simulink model "chap04_CA1"  (R2021a)
settings: Solver=FixedStepDiscrete  StartTime=0.0  StopTime=30  FixedStep=0.001  RelTol=1e-3
undefined symbols (not defined in the file): DiscIntNeverNeededParam
libraries: simulink x4
(part 4 of 4)

== system chap04_CA1/Subsystem/Subsystem13/Subsystem7/Subsystem12 ==
  xx2 : Inport
  xx1 : Inport  Port=2
  xx4 : Inport  Port=3
  xx6 : Inport  Port=4
  Add1 : Sum  Inputs=-+
  Add2 : Sum  Inputs=+-
  Add4 : Sum  Inputs=-+
  Add5 : Sum  Inputs=+++
  Constant3 : Constant  Value=0.5
  Constant4 : Constant  Value=1.0
  Constant5 : Constant  Value=1.5
  Product3 : Product
  Product4 : Product
  Product5 : Product
  p2x : Outport
  wires:
  Product4/1 -> Add5/2
  Product5/1 -> Add5/3
  Constant3/1 -> Product4/1
  Add4/1 -> Product4/2
  xx2/1 -> Add1/2, Add4/2, Add2/1
  Constant4/1 -> Product5/2
  Add2/1 -> Product5/1
  xx4/1 -> Add4/1
  xx1/1 -> Add2/2
  xx6/1 -> Add1/1
  Constant5/1 -> Product3/1
  Add1/1 -> Product3/2
  Product3/1 -> Add5/1
  Add5/1 -> p2x/1

== system chap04_CA1/Subsystem/Subsystem13/Subsystem7/Subsystem7 ==
  vy2 : Inport
  vy1 : Inport  Port=2
  vy4 : Inport  Port=3
  vy6 : Inport  Port=4
  Add6 : Sum  Inputs=-+
  Add7 : Sum  Inputs=+-
  Add8 : Sum  Inputs=-+
  Add9 : Sum  Inputs=+++
  Constant3 : Constant  Value=0.5
  Constant4 : Constant  Value=1.0
  Constant5 : Constant  Value=1.5
  Product7 : Product
  Product8 : Product
  Product9 : Product
  p2y : Outport
  wires:
  Product8/1 -> Add9/2
  Product9/1 -> Add9/3
  Constant3/1 -> Product8/1
  Add8/1 -> Product8/2
  vy2/1 -> Add6/2, Add8/2, Add7/1
  Constant4/1 -> Product9/2
  Add7/1 -> Product9/1
  vy4/1 -> Add8/1
  vy1/1 -> Add7/2
  vy6/1 -> Add6/1
  Constant5/1 -> Product7/1
  Add6/1 -> Product7/2
  Product7/1 -> Add9/1
  Add9/1 -> p2y/1

== system chap04_CA1/Subsystem/Subsystem13/Subsystem7/Subsystem8 ==
  vz2 : Inport
  vz1 : Inport  Port=2
  vz4 : Inport  Port=3
  vz6 : Inport  Port=4
  Add6 : Sum  Inputs=-+
  Add7 : Sum  Inputs=+-
  Add8 : Sum  Inputs=-+
  Add9 : Sum  Inputs=+++
  Constant3 : Constant  Value=0.5
  Constant4 : Constant  Value=1.0
  Constant5 : Constant  Value=1.5
  Product7 : Product
  Product8 : Product
  Product9 : Product
  p2z : Outport
  wires:
  Product7/1 -> Add9/1
  Add6/1 -> Product7/2
  Constant5/1 -> Product7/1
  vz6/1 -> Add6/1
  vz1/1 -> Add7/2
  vz4/1 -> Add8/1
  Add7/1 -> Product9/1
  Constant4/1 -> Product9/2
  vz2/1 -> Add7/1, Add8/2, Add6/2
  Add8/1 -> Product8/2
  Constant3/1 -> Product8/1
  Product9/1 -> Add9/3
  Product8/1 -> Add9/2
  Add9/1 -> p2z/1

== system chap04_CA1/Subsystem/Subsystem13/Subsystem7/Subsystem9 ==
  vx2 : Inport
  vx1 : Inport  Port=2
  vx4 : Inport  Port=3
  vx6 : Inport  Port=4
  Add6 : Sum  Inputs=-+
  Add7 : Sum  Inputs=+-
  Add8 : Sum  Inputs=-+
  Add9 : Sum  Inputs=+++
  Constant3 : Constant  Value=0.5
  Constant4 : Constant  Value=1.0
  Constant5 : Constant  Value=1.5
  Product7 : Product
  Product8 : Product
  Product9 : Product
  p2x : Outport
  wires:
  Add9/1 -> p2x/1
  Product7/1 -> Add9/1
  Add6/1 -> Product7/2
  Constant5/1 -> Product7/1
  vx6/1 -> Add6/1
  vx1/1 -> Add7/2
  vx4/1 -> Add8/1
  Add7/1 -> Product9/1
  Constant4/1 -> Product9/2
  vx2/1 -> Add7/1, Add8/2, Add6/2
  Add8/1 -> Product8/2
  Constant3/1 -> Product8/1
  Product9/1 -> Add9/3
  Product8/1 -> Add9/2

== system chap04_CA1/Subsystem/Subsystem6/Subsystem/Subsystem3 ==
  xyk : Inport
  xy : Inport  Port=2
  Add4 : Sum  Inputs=-+
  exy : Outport
  wires:
  xy/1 -> Add4/1
  Add4/1 -> exy/1
  xyk/1 -> Add4/2

== system chap04_CA1/Subsystem/Subsystem6/Subsystem/Subsystem4 ==
  xzk : Inport
  xz : Inport  Port=2
  Add4 : Sum  Inputs=-+
  exz : Outport
  wires:
  xzk/1 -> Add4/2
  Add4/1 -> exz/1
  xz/1 -> Add4/1

== system chap04_CA1/Subsystem/Subsystem6/Subsystem/Subsystem5 ==
  xxk : Inport
  xx : Inport  Port=2
  Add4 : Sum  Inputs=-+
  exx : Outport
  wires:
  xxk/1 -> Add4/2
  Add4/1 -> exx/1
  xx/1 -> Add4/1

== system chap04_CA1/Subsystem/Subsystem6/Subsystem/Subsystem7 ==
  vyk : Inport
  vy : Inport  Port=2
  Add8 : Sum  Inputs=-+
  ey : Outport
  wires:
  Add8/1 -> ey/1
  vy/1 -> Add8/1
  vyk/1 -> Add8/2

== system chap04_CA1/Subsystem/Subsystem6/Subsystem/Subsystem8 ==
  vzk : Inport
  vz : Inport  Port=2
  Add8 : Sum  Inputs=-+
  ez : Outport
  wires:
  vzk/1 -> Add8/2
  vz/1 -> Add8/1
  Add8/1 -> ez/1

== system chap04_CA1/Subsystem/Subsystem6/Subsystem/Subsystem9 ==
  vxk : Inport
  vx : Inport  Port=2
  Add8 : Sum  Inputs=-+
  evx : Outport
  wires:
  vxk/1 -> Add8/2
  vx/1 -> Add8/1
  Add8/1 -> evx/1

== system chap04_CA1/Subsystem/Subsystem6/Subsystem7/Subsystem1 ==
  xy1 : Inport
  xy2 : Inport  Port=2
  xy3 : Inport  Port=3
  xy6 : Inport  Port=4
  Add1 : Sum  Inputs=-+
  Add2 : Sum  Inputs=+-
  Add4 : Sum  Inputs=-+
  Add5 : Sum  Inputs=+++
  Constant1 : Constant  Value=0.5
  Constant2 : Constant  Value=1.0
  Constant6 : Constant  Value=1.2
  Product3 : Product
  Product4 : Product
  Product5 : Product
  pxy : Outport
  wires:
  Product4/1 -> Add5/2
  Product5/1 -> Add5/3
  Constant1/1 -> Product4/1
  Add4/1 -> Product4/2
  xy1/1 -> Add1/2, Add4/2, Add2/1
  Constant2/1 -> Product5/2
  Add2/1 -> Product5/1
  Add5/1 -> pxy/1
  xy3/1 -> Add4/1
  xy2/1 -> Add2/2
  xy6/1 -> Add1/1
  Constant6/1 -> Product3/1
  Add1/1 -> Product3/2
  Product3/1 -> Add5/1

== system chap04_CA1/Subsystem/Subsystem6/Subsystem7/Subsystem2 ==
  xz1 : Inport
  xx2 : Inport  Port=2
  xz3 : Inport  Port=3
  xz6 : Inport  Port=4
  Add1 : Sum  Inputs=-+
  Add2 : Sum  Inputs=+-
  Add4 : Sum  Inputs=-+
  Add5 : Sum  Inputs=+++
  Constant1 : Constant  Value=0.5
  Constant2 : Constant  Value=1.0
  Constant6 : Constant  Value=1.2
  Product3 : Product
  Product4 : Product
  Product5 : Product
  pxz : Outport
  wires:
  Product3/1 -> Add5/1
  Add1/1 -> Product3/2
  Constant6/1 -> Product3/1
  xz6/1 -> Add1/1
  xx2/1 -> Add2/2
  xz3/1 -> Add4/1
  Add5/1 -> pxz/1
  Add2/1 -> Product5/1
  Constant2/1 -> Product5/2
  xz1/1 -> Add2/1, Add4/2, Add1/2
  Add4/1 -> Product4/2
  Constant1/1 -> Product4/1
  Product5/1 -> Add5/3
  Product4/1 -> Add5/2

== system chap04_CA1/Subsystem/Subsystem6/Subsystem7/Subsystem3 ==
  vy1 : Inport
  vy2 : Inport  Port=2
  vy3 : Inport  Port=3
  vy6 : Inport  Port=4
  Add6 : Sum  Inputs=-+
  Add7 : Sum  Inputs=+-
  Add8 : Sum  Inputs=-+
  Add9 : Sum  Inputs=+++
  Constant1 : Constant  Value=0.5
  Constant2 : Constant  Value=1.0
  Constant6 : Constant  Value=1.2
  Product7 : Product
  Product8 : Product
  Product9 : Product
  pvy : Outport
  wires:
  Product8/1 -> Add9/2
  Product9/1 -> Add9/3
  Constant1/1 -> Product8/1
  Add8/1 -> Product8/2
  vy1/1 -> Add6/2, Add8/2, Add7/1
  Constant2/1 -> Product9/2
  Add7/1 -> Product9/1
  vy3/1 -> Add8/1
  vy2/1 -> Add7/2
  vy6/1 -> Add6/1
  Constant6/1 -> Product7/1
  Add6/1 -> Product7/2
  Product7/1 -> Add9/1
  Add9/1 -> pvy/1

== system chap04_CA1/Subsystem/Subsystem6/Subsystem7/Subsystem4 ==
  vz1 : Inport
  vz2 : Inport  Port=2
  vz3 : Inport  Port=3
  vz6 : Inport  Port=4
  Add6 : Sum  Inputs=-+
  Add7 : Sum  Inputs=+-
  Add8 : Sum  Inputs=-+
  Add9 : Sum  Inputs=+++
  Constant1 : Constant  Value=0.5
  Constant2 : Constant  Value=1.0
  Constant6 : Constant  Value=1.2
  Product7 : Product
  Product8 : Product
  Product9 : Product
  pvz : Outport
  wires:
  Add9/1 -> pvz/1
  Product7/1 -> Add9/1
  Add6/1 -> Product7/2
  Constant6/1 -> Product7/1
  vz6/1 -> Add6/1
  vz2/1 -> Add7/2
  vz3/1 -> Add8/1
  Add7/1 -> Product9/1
  Constant2/1 -> Product9/2
  vz1/1 -> Add7/1, Add8/2, Add6/2
  Add8/1 -> Product8/2
  Constant1/1 -> Product8/1
  Product9/1 -> Add9/3
  Product8/1 -> Add9/2

== system chap04_CA1/Subsystem/Subsystem6/Subsystem7/Subsystem5 ==
  vx1 : Inport
  vx2 : Inport  Port=2
  vx3 : Inport  Port=3
  vx6 : Inport  Port=4
  Add6 : Sum  Inputs=-+
  Add7 : Sum  Inputs=+-
  Add8 : Sum  Inputs=-+
  Add9 : Sum  Inputs=+++
  Constant1 : Constant  Value=0.5
  Constant2 : Constant  Value=1.0
  Constant6 : Constant  Value=1.2
  Product7 : Product
  Product8 : Product
  Product9 : Product
  pvx : Outport
  wires:
  Add9/1 -> pvx/1
  Product7/1 -> Add9/1
  Add6/1 -> Product7/2
  Constant6/1 -> Product7/1
  vx6/1 -> Add6/1
  vx2/1 -> Add7/2
  vx3/1 -> Add8/1
  Add7/1 -> Product9/1
  Constant2/1 -> Product9/2
  vx1/1 -> Add7/1, Add8/2, Add6/2
  Add8/1 -> Product8/2
  Constant1/1 -> Product8/1
  Product9/1 -> Add9/3
  Product8/1 -> Add9/2

== system chap04_CA1/Subsystem/Subsystem6/Subsystem7/Subsystem6 ==
  xx1 : Inport
  xx2 : Inport  Port=2
  xx3 : Inport  Port=3
  xx6 : Inport  Port=4
  Add1 : Sum  Inputs=-+
  Add2 : Sum  Inputs=+-
  Add4 : Sum  Inputs=-+
  Add5 : Sum  Inputs=+++
  Constant1 : Constant  Value=0.5
  Constant2 : Constant  Value=1.0
  Constant6 : Constant  Value=1.2
  Product3 : Product
  Product4 : Product
  Product5 : Product
  pxx : Outport
  wires:
  Product3/1 -> Add5/1
  Add1/1 -> Product3/2
  Constant6/1 -> Product3/1
  xx6/1 -> Add1/1
  xx2/1 -> Add2/2
  xx3/1 -> Add4/1
  Add2/1 -> Product5/1
  Constant2/1 -> Product5/2
  xx1/1 -> Add2/1, Add4/2, Add1/2
  Add4/1 -> Product4/2
  Constant1/1 -> Product4/1
  Product5/1 -> Add5/3
  Product4/1 -> Add5/2
  Add5/1 -> pxx/1

== system chap04_CA1/Subsystem/Subsystem7/Subsystem7/Subsystem3 ==
  xyk : Inport
  xy : Inport  Port=2
  Add4 : Sum  Inputs=-+
  exy : Outport
  wires:
  xy/1 -> Add4/1
  Add4/1 -> exy/1
  xyk/1 -> Add4/2

== system chap04_CA1/Subsystem/Subsystem7/Subsystem7/Subsystem4 ==
  xzk : Inport
  xz : Inport  Port=2
  Add4 : Sum  Inputs=-+
  exz : Outport
  wires:
  xzk/1 -> Add4/2
  Add4/1 -> exz/1
  xz/1 -> Add4/1

== system chap04_CA1/Subsystem/Subsystem7/Subsystem7/Subsystem5 ==
  xxk : Inport
  xx : Inport  Port=2
  Add4 : Sum  Inputs=-+
  exx : Outport
  wires:
  xxk/1 -> Add4/2
  Add4/1 -> exx/1
  xx/1 -> Add4/1

== system chap04_CA1/Subsystem/Subsystem7/Subsystem7/Subsystem7 ==
  vyk : Inport
  vy : Inport  Port=2
  Add8 : Sum  Inputs=-+
  ey : Outport
  wires:
  Add8/1 -> ey/1
  vy/1 -> Add8/1
  vyk/1 -> Add8/2

== system chap04_CA1/Subsystem/Subsystem7/Subsystem7/Subsystem8 ==
  vzk : Inport
  vz : Inport  Port=2
  Add8 : Sum  Inputs=-+
  ez : Outport
  wires:
  vzk/1 -> Add8/2
  vz/1 -> Add8/1
  Add8/1 -> ez/1

== system chap04_CA1/Subsystem/Subsystem7/Subsystem7/Subsystem9 ==
  vxk : Inport
  vx : Inport  Port=2
  Add8 : Sum  Inputs=-+
  evx : Outport
  wires:
  vxk/1 -> Add8/2
  vx/1 -> Add8/1
  Add8/1 -> evx/1

== system chap04_CA1/Subsystem/Subsystem7/Subsystem8/Subsystem1 ==
  vy5 : Inport
  vy0 : Inport  Port=2
  Add6 : Sum  Inputs=+-
  Constant7 : Constant  Value=2.0
  Product7 : Product
  uty : Outport
  wires:
  vy0/1 -> Add6/2
  Constant7/1 -> Product7/2
  Add6/1 -> Product7/1
  Product7/1 -> uty/1
  vy5/1 -> Add6/1

== system chap04_CA1/Subsystem/Subsystem7/Subsystem8/Subsystem10 ==
  xy5 : Inport
  xy0 : Inport  Port=2
  Add1 : Sum  Inputs=-+
  Constant7 : Constant  Value=2.0
  Product3 : Product
  uty : Outport
  wires:
  xy0/1 -> Add1/1
  Add1/1 -> Product3/2
  Constant7/1 -> Product3/1
  xy5/1 -> Add1/2
  Product3/1 -> uty/1

== system chap04_CA1/Subsystem/Subsystem7/Subsystem8/Subsystem11 ==
  xz5 : Inport
  xz0 : Inport  Port=2
  Add1 : Sum  Inputs=-+
  Constant7 : Constant  Value=2.0
  Product3 : Product
  utz : Outport
  wires:
  Product3/1 -> utz/1
  xz5/1 -> Add1/2
  Constant7/1 -> Product3/1
  Add1/1 -> Product3/2
  xz0/1 -> Add1/1

== system chap04_CA1/Subsystem/Subsystem7/Subsystem8/Subsystem12 ==
  xx5 : Inport
  xx0 : Inport  Port=2
  Add1 : Sum  Inputs=-+
  Constant7 : Constant  Value=2.0
  Product3 : Product
  utx : Outport
  wires:
  Product3/1 -> utx/1
  xx5/1 -> Add1/2
  Constant7/1 -> Product3/1
  Add1/1 -> Product3/2
  xx0/1 -> Add1/1

== system chap04_CA1/Subsystem/Subsystem7/Subsystem8/Subsystem2 ==
  vy5 : Inport
  vy3 : Inport  Port=2
  vy4 : Inport  Port=3
  Add10 : Sum  Inputs=-+
  Add8 : Sum
  Add9 : Sum  Inputs=+-
  Constant1 : Constant  Value=1.2
  Constant2 : Constant  Value=1.5
  Product8 : Product
  Product9 : Product
  uty : Outport
  wires:
  Product9/1 -> Add8/2
  Product8/1 -> Add8/1
  Add9/1 -> Product9/1
  Constant2/1 -> Product9/2
  Add10/1 -> Product8/2
  Constant1/1 -> Product8/1
  vy3/1 -> Add9/2
  vy4/1 -> Add10/1
  vy5/1 -> Add9/1, Add10/2
  Add8/1 -> uty/1

== system chap04_CA1/Subsystem/Subsystem7/Subsystem8/Subsystem3 ==
  vz5 : Inport
  vz0 : Inport  Port=2
  Add6 : Sum  Inputs=+-
  Constant7 : Constant  Value=2.0
  Product7 : Product
  utz : Outport
  wires:
  vz5/1 -> Add6/1
  Product7/1 -> utz/1
  Add6/1 -> Product7/1
  Constant7/1 -> Product7/2
  vz0/1 -> Add6/2

== system chap04_CA1/Subsystem/Subsystem7/Subsystem8/Subsystem4 ==
  vx5 : Inport
  vx0 : Inport  Port=2
  Add6 : Sum  Inputs=+-
  Constant7 : Constant  Value=2.0
  Product7 : Product
  utx : Outport
  wires:
  vx5/1 -> Add6/1
  Product7/1 -> utx/1
  Add6/1 -> Product7/1
  Constant7/1 -> Product7/2
  vx0/1 -> Add6/2

== system chap04_CA1/Subsystem/Subsystem7/Subsystem8/Subsystem5 ==
  vz5 : Inport
  vz3 : Inport  Port=2
  vz4 : Inport  Port=3
  Add10 : Sum  Inputs=-+
  Add8 : Sum
  Add9 : Sum  Inputs=+-
  Constant1 : Constant  Value=1.2
  Constant2 : Constant  Value=1.5
  Product8 : Product
  Product9 : Product
  utz : Outport
  wires:
  vz5/1 -> Add10/2, Add9/1
  vz4/1 -> Add10/1
  vz3/1 -> Add9/2
  Constant1/1 -> Product8/1
  Add10/1 -> Product8/2
  Constant2/1 -> Product9/2
  Add9/1 -> Product9/1
  Product8/1 -> Add8/1
  Product9/1 -> Add8/2
  Add8/1 -> utz/1

== system chap04_CA1/Subsystem/Subsystem7/Subsystem8/Subsystem6 ==
  vx5 : Inport
  vx3 : Inport  Port=2
  vx4 : Inport  Port=3
  Add10 : Sum  Inputs=-+
  Add8 : Sum
  Add9 : Sum  Inputs=+-
  Constant1 : Constant  Value=1.2
  Constant2 : Constant  Value=1.5
  Product8 : Product
  Product9 : Product
  utx : Outport
  wires:
  vx5/1 -> Add10/2, Add9/1
  vx4/1 -> Add10/1
  vx3/1 -> Add9/2
  Add8/1 -> utx/1
  Constant1/1 -> Product8/1
  Add10/1 -> Product8/2
  Constant2/1 -> Product9/2
  Add9/1 -> Product9/1
  Product8/1 -> Add8/1
  Product9/1 -> Add8/2

== system chap04_CA1/Subsystem/Subsystem7/Subsystem8/Subsystem7 ==
  xy5 : Inport
  xy3 : Inport  Port=2
  xy4 : Inport  Port=3
  Add2 : Sum  Inputs=+-
  Add4 : Sum  Inputs=-+
  Add5 : Sum
  Constant1 : Constant  Value=1.2
  Constant2 : Constant  Value=1.5
  Product4 : Product
  Product5 : Product
  uty : Outport
  wires:
  Product4/1 -> Add5/1
  Product5/1 -> Add5/2
  Constant1/1 -> Product4/1
  Add4/1 -> Product4/2
  xy5/1 -> Add2/1, Add4/2
  Constant2/1 -> Product5/2
  Add2/1 -> Product5/1
  xy4/1 -> Add4/1
  xy3/1 -> Add2/2
  Add5/1 -> uty/1

== system chap04_CA1/Subsystem/Subsystem7/Subsystem8/Subsystem8 ==
  xz5 : Inport
  xz3 : Inport  Port=2
  xz4 : Inport  Port=3
  Add2 : Sum  Inputs=+-
  Add4 : Sum  Inputs=-+
  Add5 : Sum
  Constant1 : Constant  Value=1.2
  Constant2 : Constant  Value=1.5
  Product4 : Product
  Product5 : Product
  utz : Outport
  wires:
  xz3/1 -> Add2/2
  xz4/1 -> Add4/1
  Add2/1 -> Product5/1
  Constant2/1 -> Product5/2
  xz5/1 -> Add4/2, Add2/1
  Add4/1 -> Product4/2
  Constant1/1 -> Product4/1
  Product5/1 -> Add5/2
  Product4/1 -> Add5/1
  Add5/1 -> utz/1

== system chap04_CA1/Subsystem/Subsystem7/Subsystem8/Subsystem9 ==
  xx5 : Inport
  xx3 : Inport  Port=2
  xx4 : Inport  Port=3
  Add2 : Sum  Inputs=+-
  Add4 : Sum  Inputs=-+
  Add5 : Sum
  Constant1 : Constant  Value=1.2
  Constant2 : Constant  Value=1.5
  Product4 : Product
  Product5 : Product
  utx : Outport
  wires:
  xx3/1 -> Add2/2
  xx4/1 -> Add4/1
  Add2/1 -> Product5/1
  Constant2/1 -> Product5/2
  xx5/1 -> Add4/2, Add2/1
  Add4/1 -> Product4/2
  Constant1/1 -> Product4/1
  Product5/1 -> Add5/2
  Add5/1 -> utx/1
  Product4/1 -> Add5/1

== system chap04_CA1/Subsystem/Subsystem9/Subsystem7/Subsystem3 ==
  xyk : Inport
  xy : Inport  Port=2
  Add4 : Sum  Inputs=-+
  exy : Outport
  wires:
  xy/1 -> Add4/1
  Add4/1 -> exy/1
  xyk/1 -> Add4/2

== system chap04_CA1/Subsystem/Subsystem9/Subsystem7/Subsystem4 ==
  xzk : Inport
  xz : Inport  Port=2
  Add4 : Sum  Inputs=-+
  exz : Outport
  wires:
  xzk/1 -> Add4/2
  Add4/1 -> exz/1
  xz/1 -> Add4/1

== system chap04_CA1/Subsystem/Subsystem9/Subsystem7/Subsystem5 ==
  xxk : Inport
  xx : Inport  Port=2
  Add4 : Sum  Inputs=-+
  exx : Outport
  wires:
  xxk/1 -> Add4/2
  Add4/1 -> exx/1
  xx/1 -> Add4/1

== system chap04_CA1/Subsystem/Subsystem9/Subsystem7/Subsystem7 ==
  vyk : Inport
  vy : Inport  Port=2
  Add8 : Sum  Inputs=-+
  ey : Outport
  wires:
  Add8/1 -> ey/1
  vy/1 -> Add8/1
  vyk/1 -> Add8/2

== system chap04_CA1/Subsystem/Subsystem9/Subsystem7/Subsystem8 ==
  vzk : Inport
  vz : Inport  Port=2
  Add8 : Sum  Inputs=-+
  ez : Outport
  wires:
  vzk/1 -> Add8/2
  vz/1 -> Add8/1
  Add8/1 -> ez/1

== system chap04_CA1/Subsystem/Subsystem9/Subsystem7/Subsystem9 ==
  vxk : Inport
  vx : Inport  Port=2
  Add8 : Sum  Inputs=-+
  evx : Outport
  wires:
  vxk/1 -> Add8/2
  vx/1 -> Add8/1
  Add8/1 -> evx/1

== system chap04_CA1/Subsystem/Subsystem9/Subsystem8/Subsystem10 ==
  xy3 : Inport
  xy1 : Inport  Port=2
  xy4 : Inport  Port=3
  xy5 : Inport  Port=4
  Add1 : Sum  Inputs=-+
  Add2 : Sum  Inputs=+-
  Add4 : Sum  Inputs=-+
  Add5 : Sum  Inputs=+++
  Constant3 : Constant  Value=1.0
  Constant4 : Constant  Value=0.5
  Constant5 : Constant  Value=1.5
  Product3 : Product
  Product4 : Product
  Product5 : Product
  p3y : Outport
  wires:
  Product4/1 -> Add5/2
  Product5/1 -> Add5/3
  Constant3/1 -> Product4/1
  Add4/1 -> Product4/2
  xy3/1 -> Add1/2, Add4/2, Add2/1
  Constant4/1 -> Product5/2
  Add2/1 -> Product5/1
  xy4/1 -> Add4/1
  xy1/1 -> Add2/2
  xy5/1 -> Add1/1
  Constant5/1 -> Product3/1
  Add1/1 -> Product3/2
  Product3/1 -> Add5/1
  Add5/1 -> p3y/1

== system chap04_CA1/Subsystem/Subsystem9/Subsystem8/Subsystem11 ==
  xz3 : Inport
  xz1 : Inport  Port=2
  xz4 : Inport  Port=3
  xz5 : Inport  Port=4
  Add1 : Sum  Inputs=-+
  Add2 : Sum  Inputs=+-
  Add4 : Sum  Inputs=-+
  Add5 : Sum  Inputs=+++
  Constant3 : Constant  Value=1.0
  Constant4 : Constant  Value=0.5
  Constant5 : Constant  Value=1.5
  Product3 : Product
  Product4 : Product
  Product5 : Product
  p3z : Outport
  wires:
  Product3/1 -> Add5/1
  Add1/1 -> Product3/2
  Constant5/1 -> Product3/1
  xz5/1 -> Add1/1
  xz1/1 -> Add2/2
  xz4/1 -> Add4/1
  Add2/1 -> Product5/1
  Constant4/1 -> Product5/2
  xz3/1 -> Add2/1, Add4/2, Add1/2
  Add4/1 -> Product4/2
  Constant3/1 -> Product4/1
  Product5/1 -> Add5/3
  Product4/1 -> Add5/2
  Add5/1 -> p3z/1

== system chap04_CA1/Subsystem/Subsystem9/Subsystem8/Subsystem12 ==
  xx3 : Inport
  xx1 : Inport  Port=2
  xx4 : Inport  Port=3
  xx5 : Inport  Port=4
  Add1 : Sum  Inputs=-+
  Add2 : Sum  Inputs=+-
  Add4 : Sum  Inputs=-+
  Add5 : Sum  Inputs=+++
  Constant3 : Constant  Value=1.0
  Constant4 : Constant  Value=0.5
  Constant5 : Constant  Value=1.5
  Product3 : Product
  Product4 : Product
  Product5 : Product
  p3x : Outport
  wires:
  Product3/1 -> Add5/1
  Add1/1 -> Product3/2
  Constant5/1 -> Product3/1
  xx5/1 -> Add1/1
  xx1/1 -> Add2/2
  xx4/1 -> Add4/1
  Add5/1 -> p3x/1
  Add2/1 -> Product5/1
  Constant4/1 -> Product5/2
  xx3/1 -> Add2/1, Add4/2, Add1/2
  Add4/1 -> Product4/2
  Constant3/1 -> Product4/1
  Product5/1 -> Add5/3
  Product4/1 -> Add5/2

== system chap04_CA1/Subsystem/Subsystem9/Subsystem8/Subsystem7 ==
  vy3 : Inport
  vy1 : Inport  Port=2
  vy4 : Inport  Port=3
  vy5 : Inport  Port=4
  Add6 : Sum  Inputs=-+
  Add7 : Sum  Inputs=+-
  Add8 : Sum  Inputs=-+
  Add9 : Sum  Inputs=+++
  Constant3 : Constant  Value=1.0
  Constant4 : Constant  Value=0.5
  Constant5 : Constant  Value=1.5
  Product7 : Product
  Product8 : Product
  Product9 : Product
  p3y : Outport
  wires:
  Product7/1 -> Add9/1
  Add6/1 -> Product7/2
  Constant5/1 -> Product7/1
  vy5/1 -> Add6/1
  vy1/1 -> Add7/2
  vy4/1 -> Add8/1
  Add7/1 -> Product9/1
  Constant4/1 -> Product9/2
  vy3/1 -> Add7/1, Add8/2, Add6/2
  Add8/1 -> Product8/2
  Constant3/1 -> Product8/1
  Product9/1 -> Add9/3
  Product8/1 -> Add9/2
  Add9/1 -> p3y/1

== system chap04_CA1/Subsystem/Subsystem9/Subsystem8/Subsystem8 ==
  vz3 : Inport
  vz1 : Inport  Port=2
  vz4 : Inport  Port=3
  vz5 : Inport  Port=4
  Add6 : Sum  Inputs=-+
  Add7 : Sum  Inputs=+-
  Add8 : Sum  Inputs=-+
  Add9 : Sum  Inputs=+++
  Constant3 : Constant  Value=1.0
  Constant4 : Constant  Value=0.5
  Constant5 : Constant  Value=1.5
  Product7 : Product
  Product8 : Product
  Product9 : Product
  p3z : Outport
  wires:
  Product8/1 -> Add9/2
  Product9/1 -> Add9/3
  Constant3/1 -> Product8/1
  Add8/1 -> Product8/2
  vz3/1 -> Add6/2, Add8/2, Add7/1
  Constant4/1 -> Product9/2
  Add7/1 -> Product9/1
  vz4/1 -> Add8/1
  vz1/1 -> Add7/2
  vz5/1 -> Add6/1
  Constant5/1 -> Product7/1
  Add6/1 -> Product7/2
  Product7/1 -> Add9/1
  Add9/1 -> p3z/1

== system chap04_CA1/Subsystem/Subsystem9/Subsystem8/Subsystem9 ==
  vx3 : Inport
  vx1 : Inport  Port=2
  vx4 : Inport  Port=3
  vx5 : Inport  Port=4
  Add6 : Sum  Inputs=-+
  Add7 : Sum  Inputs=+-
  Add8 : Sum  Inputs=-+
  Add9 : Sum  Inputs=+++
  Constant3 : Constant  Value=1.0
  Constant4 : Constant  Value=0.5
  Constant5 : Constant  Value=1.5
  Product7 : Product
  Product8 : Product
  Product9 : Product
  p3x : Outport
  wires:
  Product8/1 -> Add9/2
  Product9/1 -> Add9/3
  Constant3/1 -> Product8/1
  Add8/1 -> Product8/2
  vx3/1 -> Add6/2, Add8/2, Add7/1
  Constant4/1 -> Product9/2
  Add7/1 -> Product9/1
  vx4/1 -> Add8/1
  vx1/1 -> Add7/2
  vx5/1 -> Add6/1
  Constant5/1 -> Product7/1
  Add6/1 -> Product7/2
  Product7/1 -> Add9/1
  Add9/1 -> p3x/1

== matlab function chap04_CA1/Subsystem/Subsystem6/Subsystem/MATLAB Function1 ==
  data: u input; y output
function y = fcn(u)

y = norm(u);

== matlab function chap04_CA1/Subsystem/Subsystem11/Subsystem7/MATLAB Function1 ==
  data: u input; y output
function y = fcn(u)

y = norm(u);

== matlab function chap04_CA1/Subsystem/Subsystem11/Subsystem7/MATLAB Function2 ==
  data: u input; y output
function y = fcn(u)

y = norm(u);

== matlab function chap04_CA1/Subsystem/Subsystem11/Subsystem8/MATLAB Function2 ==
  data: u input; y output
function y = fcn(u)

y = norm(u);

== matlab function chap04_CA1/Subsystem/Subsystem7/Subsystem7/MATLAB Function1 ==
  data: u input; y output
function y = fcn(u)

y = norm(u);

== matlab function chap04_CA1/Subsystem/Subsystem13/Subsystem3/MATLAB Function1 ==
  data: u input; y output
function y = fcn(u)

y = norm(u);

== matlab function chap04_CA1/Subsystem/Subsystem7/Subsystem7/MATLAB Function2 ==
  data: u input; y output
function y = fcn(u)

y = norm(u);

== matlab function chap04_CA1/Subsystem/Subsystem11/Subsystem8/MATLAB Function4 ==
  data: u input; y output
function y = fcn(u)

y = norm(u);

== matlab function chap04_CA1/Subsystem/Subsystem6/Subsystem/MATLAB Function2 ==
  data: u input; y output
function y = fcn(u)

y = norm(u);

== matlab function chap04_CA1/Subsystem/Subsystem6/Subsystem7/MATLAB Function ==
  data: u input; y output
function y = fcn(u)

y = norm(u);

== matlab function chap04_CA1/Subsystem/Subsystem6/Subsystem7/MATLAB Function1 ==
  data: u input; y output
function y = fcn(u)

y = norm(u);

== matlab function chap04_CA1/Subsystem/Subsystem9/Subsystem8/MATLAB Function ==
  data: u input; y output
function y = fcn(u)

y = norm(u);

== matlab function chap04_CA1/Subsystem/Subsystem9/Subsystem7/MATLAB Function2 ==
  data: u input; y output
function y = fcn(u)

y = norm(u);

== matlab function chap04_CA1/Subsystem/Subsystem11/Subsystem8/MATLAB Function5 ==
  data: u input; y output
function y = fcn(u)

y = norm(u);

== matlab function chap04_CA1/Subsystem/Subsystem9/Subsystem8/MATLAB Function1 ==
  data: u input; y output
function y = fcn(u)

y = norm(u);

== matlab function chap04_CA1/Subsystem/Subsystem13/Subsystem3/MATLAB Function2 ==
  data: u input; y output
function y = fcn(u)

y = norm(u);

== matlab function chap04_CA1/Subsystem/Subsystem10/Subsystem8/MATLAB Function1 ==
  data: u input; y output
function y = fcn(u)

y = norm(u);

== matlab function chap04_CA1/Subsystem/Subsystem9/Subsystem7/MATLAB Function1 ==
  data: u input; y output
function y = fcn(u)

y = norm(u);

== matlab function chap04_CA1/Subsystem/Subsystem7/Subsystem8/MATLAB Function4 ==
  data: u input; y output
function y = fcn(u)

y = norm(u);

== matlab function chap04_CA1/Subsystem/Subsystem7/Subsystem8/MATLAB Function5 ==
  data: u input; y output
function y = fcn(u)

y = norm(u);

== matlab function chap04_CA1/Subsystem/Subsystem7/Subsystem8/MATLAB Function1 ==
  data: u input; y output
function y = fcn(u)

y = norm(u);

== matlab function chap04_CA1/Subsystem/Subsystem7/Subsystem8/MATLAB Function2 ==
  data: u input; y output
function y = fcn(u)

y = norm(u);

== matlab function chap04_CA1/Subsystem/Subsystem10/Subsystem8/MATLAB Function ==
  data: u input; y output
function y = fcn(u)

y = norm(u);

== matlab function chap04_CA1/Subsystem/Subsystem10/Subsystem7/MATLAB Function1 ==
  data: u input; y output
function y = fcn(u)

y = norm(u);

== matlab function chap04_CA1/Subsystem/Subsystem10/Subsystem7/MATLAB Function2 ==
  data: u input; y output
function y = fcn(u)

y = norm(u);

== matlab function chap04_CA1/Subsystem/Subsystem11/Subsystem8/MATLAB Function1 ==
  data: u input; y output
function y = fcn(u)

y = norm(u);

== matlab function chap04_CA1/Subsystem/Subsystem13/Subsystem7/MATLAB Function ==
  data: u input; y output
function y = fcn(u)

y = norm(u);

== matlab function chap04_CA1/Subsystem/Subsystem13/Subsystem7/MATLAB Function1 ==
  data: u input; y output
function y = fcn(u)

y = norm(u);
